simulink model "active_suspension_kalman_sim"  (R2020a)
settings: Solver=ode45  StartTime=0.0  StopTime=20.0  MaxStep=0.001  RelTol=1e-3  EnableMultiTasking=on
InitFcn:
  | active_suspension_kalman_design
undefined symbols (not defined in the file): A, B1, B2, C, C1, D1
settings Model: Creator=JonasMac  LastModifiedBy=rizwanahmed
settings DataIOCC: LimitDataPoints=on  SaveFormat=Array  ReturnWorkspaceOutputs=off
settings OptimizationCC: LifeSpan=inf
settings DebuggingCC: UnderspecifiedInitializationDetection=Classic  MergeDetectMultiDrivingBlocksExec=none  SolverPrmCheckMsg=warning  SFUnexpectedBacktrackingDiag=warning  SFNoUnconditionalDefaultTransitionDiag=warning  SFExecutionAtInitializationDiag=none  ArithmeticOperatorsInVariantConditions=warning
settings HardwareCC: ProdBitPerPointer=32  ProdBitPerSizeT=32  ProdBitPerPtrDiffT=32  ProdLargestAtomicFloat=None  ProdIntDivRoundTo=Undefined  ProdEndianess=Unspecified  ProdWordSize=32  ProdHWDeviceType=32-bit Generic
settings ModelReferenceCC: PropagateSignalLabelsOutOfModel=off
settings SFSimCC: SimUseLocalCustomCode=off  CustomCodeUndefinedFunction=UseInterfaceOnly
settings RTWCC: RTWUseLocalCustomCode=off
settings CodeAppCC: StateflowObjectComments=on
settings GRTTargetCC: TargetLangStandard=C89/C90 (ANSI)
settings ConfigComp: CovMetricSettings=dw  CovHtmlReporting=on  CovSaveCumulativeToWorkspaceVar=on  CovSaveSingleToWorkspaceVar=on  CovExternalEMLEnable=off

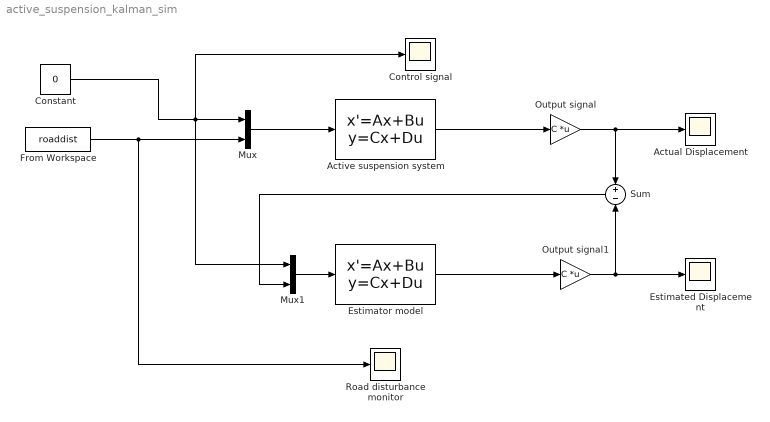
== system active_suspension_kalman_sim ==
  Active suspension system : StateSpace  A=A  B=B1  C=C1  D=D1  InitialCondition=0
  Actual Displacement : Scope
  Constant : Constant  Value=0
  Control signal : Scope
  Estimated Displacement : Scope
  Estimator model : StateSpace  A=A  B=B2  C=C1  D=D1  InitialCondition=0
  From Workspace : FromWorkspace  VariableName=roaddist
  Mux : Mux  Inputs=2
  Mux1 : Mux  Inputs=2
  Output signal : Gain  Gain=C  Multiplication=Matrix(K*u)
  Output signal1 : Gain  Gain=C  Multiplication=Matrix(K*u)
  Road disturbance monitor : Scope
  Sum : Sum  Inputs=+|-
  wires:
  Output signal/1 -> Actual Displacement/1, Sum/1
  Active suspension system/1 -> Output signal/1
  Mux/1 -> Active suspension system/1
  From Workspace/1 -> Mux/2, Road disturbance monitor/1
  Output signal1/1 -> Sum/2, Estimated Displacement/1
  Mux1/1 -> Estimator model/1
  Estimator model/1 -> Output signal1/1
  Sum/1 -> Mux1/2
  Constant/1 -> Control signal/1, Mux1/1, Mux/1
